simulink model "SoCManagement"  (R2020a)
settings: Solver=FixedStepAuto  StartTime=0.0  StopTime=200  FixedStep=1  RelTol=1e-3
libraries: ESSLibrary x1
settings Model: Creator=soumyakantapanda  LastModifiedBy=soumyakantapanda

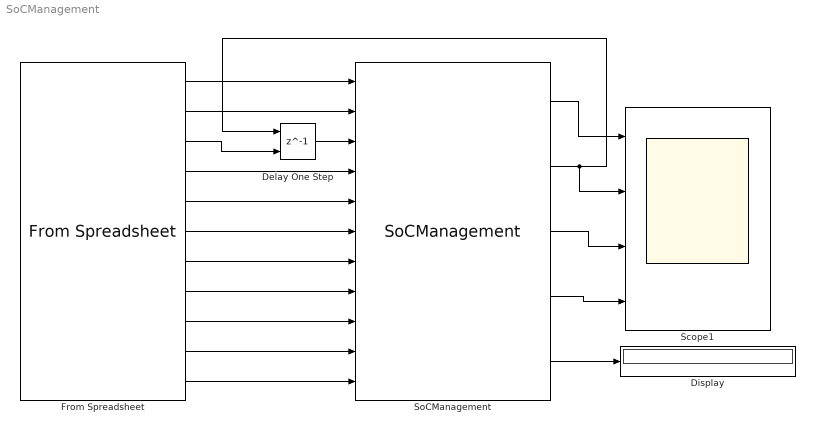
== system SoCManagement ==
  Delay One Step : Delay  DelayLength=1  InitialConditionSource=Input port
      settings: InputPortMap=u0,p4
  Display : Display
  From Spreadsheet : FromSpreadsheet  FileName=C:\Users\soumyakantapanda\OneDrive - L&T Construction\Desktop\LaptopChange\Desktop\ESS_Development\Implementation\NewDevelopment\test\SoCManagementInput.xlsx  Range=A2:L18  ExtrapolationBeforeFirstDataPoint=Ground value  InterpolationWithinTimeRange=Zero order hold  ExtrapolationAfterLastDataPoint=Hold last value
  Scope1 : Scope  NumInputPorts=4
  SoCManagement : ESSLibrary/SoCManagement  SystemSampleTime=-1  Latency=0  AutoFrameSizeCalculation=off
  wires:
  From Spreadsheet/1 -> SoCManagement/1
  From Spreadsheet/2 -> SoCManagement/2
  From Spreadsheet/4 -> SoCManagement/4
  From Spreadsheet/5 -> SoCManagement/5
  From Spreadsheet/6 -> SoCManagement/6
  From Spreadsheet/7 -> SoCManagement/7
  From Spreadsheet/8 -> SoCManagement/8
  From Spreadsheet/9 -> SoCManagement/9
  From Spreadsheet/10 -> SoCManagement/10
  From Spreadsheet/11 -> SoCManagement/11
  Delay One Step/1 -> SoCManagement/3
  SoCManagement/2 -> Scope1/2, Delay One Step/1
  From Spreadsheet/3 -> Delay One Step/2
  SoCManagement/5 -> Display/1
  SoCManagement/1 -> Scope1/1
  SoCManagement/3 -> Scope1/3
  SoCManagement/4 -> Scope1/4
